simulink model "LQR"  (R2024b)
settings: Solver=ode45  StartTime=0.0  StopTime=10  RelTol=1e-3
values from neighbouring files (symbols this model uses):
  Beq = mot.B+(mld.Bh)/((gbox.N)^2)    [LQR_code.m]
  deltafil = 2^(-0.5)    (= 0.707106781187)    [LQR_code.m]    (also in PID_Luca.m)
  Jb = 1.4e-3    (= 0.0014)    [Elastic_parameters_estimation.m]
  K = acker(Aprime,Bprime,poles)    [LQR_code.m]
  Klqr1 = lqry(sysG,1,r2)    [LQR_code.m]
  Nu = N(5)    [LQR_code.m]
  Nx = [N(1);N(2);N(3);N(4)]    [LQR_code.m]
  omegac = 2*pi*50    (= 314.159265359)    [LQR_code.m]    (also in PID_Luca.m)
  Req = sens.curr.Rs+mot.R    [LQR_code.m]
undefined symbols (not defined in the file or in its folder): Bb, daq, degs2rpm, drv, gbox, Jeq_hat, k_drv, Ke, Kt, mot, pulse2deg, rads2rpm, rpm2rads, sens, T_drv, tau_sf
settings Model: Creator=lucag  LastModifiedBy=galeazzolu

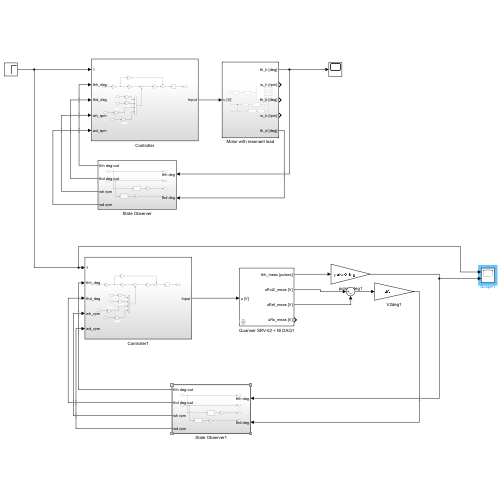
[thumbnail: Simulink's stored preview of the top-level diagram]
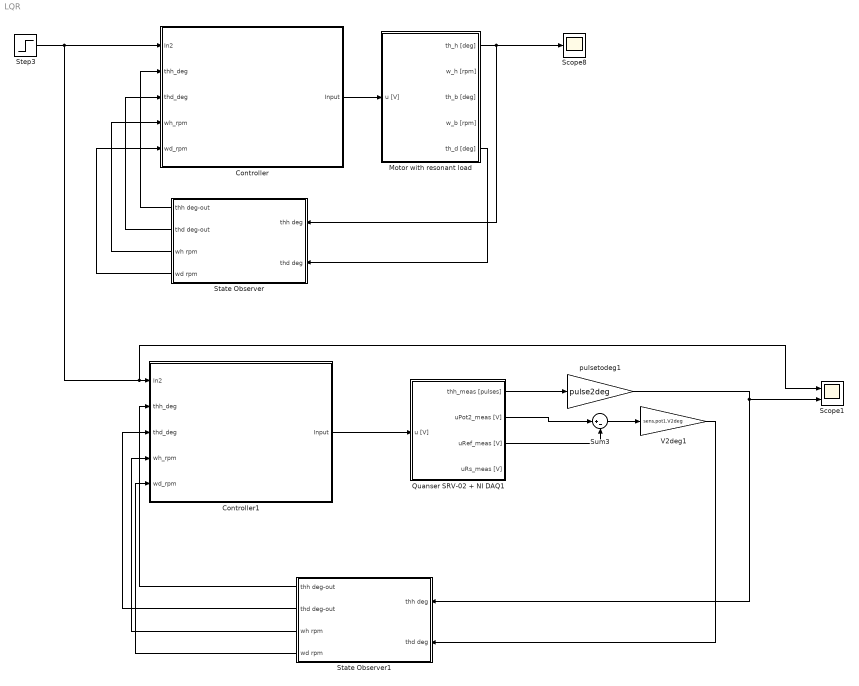
== system LQR ==
  Controller : Subsystem
  Controller1 : Subsystem
  Motor with resonant load : Subsystem
  Quanser SRV-02 + NI DAQ1 : Subsystem  mask(Quanser SRV-02 (with resonant load) + NI DAQ){Ts=0.001, fricType=Coulomb + viscous, lockShaft=off, beamInitPos=10}
      mask prompts: Ts "NI DAQ Sample Time:"; fricType "Friction model"; lockShaft "Lock motor shaft"; beamInitPos "Beam initial position [deg]:"
      mask help: Quanser SRV-02 (with resonant load) + NI DAQ model.
      mask init:
      | %%
      | % Riccardo Antonello (riccardo.antonello@unipd.it)
      | %
      | % April 28, 2020
      | %
      | % Dept. of Information Engineering, University of Padova
      | %
      | 
      | %%  Conversion gains
      | deg2rad = pi/180;                   %   [deg]   -> [rad]
      | rad2deg = 180/pi;                   %   [rad]   -> [deg]
      | 
      | 
      | %%  Sensors data
      | 
      | %   shunt resistor
      | sens.curr.Rs = 0.5;   
      | 
      | %   Hewlett-Packard HEDS-5540#A06 optical encoder
      | sens.enc.ppr = 500*4;                                                   %   pulses per rotation
      | sens.enc.pulse2deg = 360/sens.enc.ppr;                                  %   [pulses] -> [deg]
      | sens.enc.pulse2rad = 2*pi/sens.enc.ppr;                                 %   [pulses] -> [rad]
      | sens.enc.deg2pulse = sens.enc.ppr/360;                                  %   [deg] -> [pulses]
      | sens.enc.rad2pulse = sens.enc.ppr/2/pi;                                 %   [rad] -> [pulses]
      | 
      | %   potentiometer 2 (Spectrol 357-0-0-103) - installed on hub
      | sens.pot2.range.R      = 10e3;                                          %   ohmic value range 
      | sens.pot2.range.V      = 5;                                             %   voltage range
      | sens.pot2.range.th_deg = 340;                                           %   angle range [deg]
      | sens.pot2.range.th     = sens.pot2.range.th_deg * deg2rad;              %   angle range [rad]                           
      | sens.pot2.deg2V        = sens.pot2.range.V / sens.pot2.range.th_deg;    %   sensitivity [V/deg]
      | sens.pot2.rad2V        = sens.pot2.range.V / sens.pot2.range.th;        %   sensitivity [V/rad]
      | sens.pot2.V2deg        = 1/sens.pot2.deg2V;                             %   conversion gain [V] -> [deg]
      | sens.pot2.V2rad        = 1/sens.pot2.rad2V;                             %   conversion gain [V] -> [rad]
      | sens.pot2.noise.var    = 3.5e-7;                                        %   out noise variance [V^2]
      | 
      | 
      | %%  Data acquisition board (daq) data
      | 
      | %   NI PCI-6221 DAC data
      | daq.dac.bits = 16;                                  %   resolution (bits)
      | daq.dac.fs   = 10;                                  %   full scale 
      | daq.dac.q    = 2*daq.dac.fs/(2^daq.dac.bits-1);     %	quantization
      | 
      | %   NI PCI-6221 ADC data
      | daq.adc.bits = 16;                                  %   resolution (bits)
      | daq.adc.fs   = 10;                                  %   full scale (as set in SLDRT Analog Input block)
      | daq.adc.q    = 2*daq.adc.fs/(2^daq.adc.bits-1);     %   quantization   
      | 
      | 
      | %%  Set beam initial position
      | % SRV02Handle = find_system(gcb, ...
      | %     'LookUnderMasks', 'on', ...
      | %     'FindAll', 'on', ...
      | %     'FollowLinks', 'on', ...
      | %     'SearchDepth', '1', ...
      | %     'BlockType', 'ModelReference', ...
      | %     'Name', 'Quanser SRV-02');
      | %
      | % %get_param(SRV02Handle, 'InstanceParameters')
      | % InstanceParams = get_param(SRV02Handle, 'InstanceParameters');
      | % for k = 1:length(InstanceParams)
      | %     if strcmp(InstanceParams(k).Name, 'thb0')
      | %         if lockShaft
      | %             InstanceParams(k).Value = sprintf('%f', beamInitPos);
      | %         else
      | %             InstanceParams(k).Value = sprintf('%f', 0);    
      | %         end
      | %         set_param(SRV02Handle, 'InstanceParameters', InstanceParams);
      | %         break;
      | %     end
      | % end
      | 
      | if lockShaft
      |     thb0 = beamInitPos;
      | else
      |     thb0 = 0;    
      | end
      | 
      | 
      | %%  Mask initialization
      | if lockShaft
      |     
      |     %   find Inport handle
      |     InPortHandle = find_system(gcb, ...
      |         'LookUnderMasks', 'on', ...
      |         'FindAll', 'on', ...
      |         'FollowLinks', 'on', ...
      |         'SearchDepth', '1', ...
      |         'BlockType', 'Inport', ...
      |         'Name', 'u [V]');
      |     
      |     if ~isempty(InPortHandle)
      |     
      |         %   find DAC handle
      |         DACHandle = find_system(gcb, ...
      |             'LookUnderMasks', 'on', ...
      |             'FindAll', 'on', ...
      |             'FollowLinks', 'on', ...
      |             'SearchDepth', '1', ...
      |             'BlockType', 'SubSystem', ...
      |             'Name', 'DAC');  
      | 
      |         %   remove Inport output connection   
      |         InportConn = get_param(InPortHandle, 'PortConnectivity');
      |         delete_line(gcb, InportConn.Position);
      | 
      |         %   remove Inport block
      |         delete_block(InPortHandle);
      | 
      |         %   add Constant block
      |         ConstantHandle = add_block( ...
      |             'simulink/Sources/Constant', [gcb, '/u [V]'], ...
      |             'Position', [20   -37    50   -23], ...
      |             'Value', '0');
      | 
      |         %   connect Constant to DAC block
      |         DACPortHandles = get_param(DACHandle, 'PortHandles');
      |         ConstantPortHandles = get_param(ConstantHandle, 'PortHandles');
      |         add_line(gcb, ConstantPortHandles.Outport(1), DACPortHandles.Inport(1));
      |     
      |     end
      |     
      | else
      |     
      |     %   find Constant handle
      |     ConstantHandle = find_system(gcb, ...
      |         'LookUnderMasks', 'on', ...
      |         'FindAll', 'on', ...
      |         'FollowLinks', 'on', ...
      |         'SearchDepth', '1', ...
      |         'BlockType', 'Constant', ...
      |         'Name', 'u [V]');
      |     
      |     if ~isempty(ConstantHandle)
      |     
      |         %   find DAC handle
      |         DACHandle = find_system(gcb, ...
      |             'LookUnderMasks', 'on', ...
      |             'FindAll', 'on', ...
      |             'FollowLinks', 'on', ...
      |             'SearchDepth', '1', ...
      |             'BlockType', 'SubSystem', ...
      |             'Name', 'DAC');  
      |  
      |         %   remove Constant output connection   
      |         ConstantConn = get_param(ConstantHandle, 'PortConnectivity');
      |         delete_line(gcb, ConstantConn.Position);
      | 
      |         %   remove Inport block
      |         delete_block(ConstantHandle);   
      | 
      |         %   add Inport block
      |         InportHandle = add_block( ...
      |             'simulink/Sources/In1', [gcb, '/u [V]'], ...
      |             'Position', [20   -37    50   -23], ...
      |             'Port', '1');
      | 
      |         %   connect Constant to DAC block
      |         DACPortHandles = get_param(DACHandle, 'PortHandles');
      |         InportPortHandles = get_param(InportHandle, 'PortHandles');
      |         add_line(gcb, InportPortHandles.Outport(1), DACPortHandles.Inport(1));
      |     
      |      end
      |     
      | end
      mask Help:
      | Riccardo Antonello (antonello@dei.unipd.it)
      | 
      | April 28, 2020
      | 
      | Dept. of Information Engineering, University of Padova
      mask TypeOptions fricType: Coulomb + viscous | Karnopp
      mask Callback lockShaft:
      | %   get status of check box
      | lockShaft = get_param(gcb, 'lockShaft');
      | 
      | %   get current value of MaskVisibilities property
      | maskVisibilities = get_param(gcb, 'MaskVisibilities');
      | 
      | %   set visibility of the dialog box element
      | if strcmp(lockShaft, 'on')
      |     maskVisibilities{4} = 'on';
      | else
      |     maskVisibilities{4} = 'off';
      | end
      | 
      | % Set the 'MaskVisibilities' property for each parameter in mask
      | set_param( gcb, 'MaskVisibilities', maskVisibilities);
  Scope1 : Scope  NumInputPorts=2
  Scope8 : Scope
  State Observer : Subsystem
  State Observer1 : Subsystem
  Step3 : Step  Time=0  After=50  SampleTime=0.001  ZeroCross=off
  Sum3 : Sum  Inputs=|+-
  V2deg1 : Gain  Gain=sens.pot1.V2deg
  pulsetodeg1 : Gain  Gain=pulse2deg
  wires:
  Controller/1(Input) -> Motor with resonant load/1(u [V])
  Motor with resonant load/1(th_h [deg]) -> Scope8/1, State Observer/1(thh deg)
  Motor with resonant load/5(th_d [deg]) -> State Observer/2(thd deg)
  State Observer/1(thh deg-out) -> Controller/2(thh_deg)
  State Observer/2(thd deg-out) -> Controller/3(thd_deg)
  State Observer/3(wh rpm) -> Controller/4(wh_rpm)
  State Observer/4(wd rpm) -> Controller/5(wd_rpm)
  Step3/1 -> Scope1/1, Controller1/1(In2), Controller/1(In2)
  Quanser SRV-02 + NI DAQ1/3(uRef_meas [V]) -> Sum3/2
  Quanser SRV-02 + NI DAQ1/1(thh_meas [pulses]) -> pulsetodeg1/1
  Sum3/1 -> V2deg1/1
  Quanser SRV-02 + NI DAQ1/2(uPot2_meas [V]) -> Sum3/1
  pulsetodeg1/1 -> Scope1/2, State Observer1/1(thh deg)
  V2deg1/1 -> State Observer1/2(thd deg)
  State Observer1/1(thh deg-out) -> Controller1/2(thh_deg)
  State Observer1/2(thd deg-out) -> Controller1/3(thd_deg)
  State Observer1/3(wh rpm) -> Controller1/4(wh_rpm)
  State Observer1/4(wd rpm) -> Controller1/5(wd_rpm)
  Controller1/1(Input) -> Quanser SRV-02 + NI DAQ1/1(u [V])

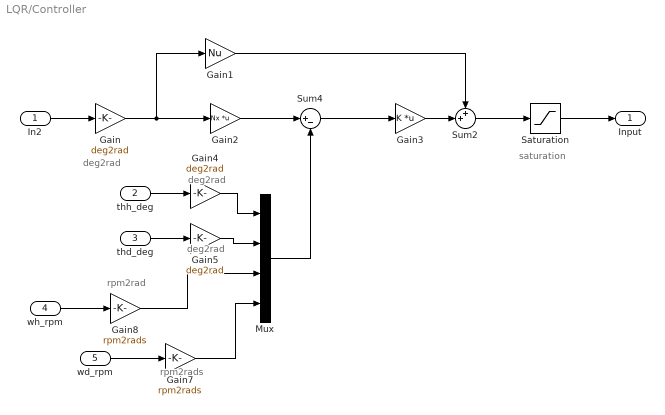
== system LQR/Controller ==
  note: rpm2rad
  note: deg2rad
  note: deg2rad
  note: deg2rad
  note: saturation
  note: rpm2rads
  In2 : Inport  PortDimensions=1
  thh_deg : Inport  Port=2
  thd_deg : Inport  Port=3
  wh_rpm : Inport  Port=4
  wd_rpm : Inport  Port=5
  Gain : Gain  Gain=deg2rad
  Gain1 : Gain  Gain=Nu
  Gain2 : Gain  Gain=Nx  Multiplication=Matrix(K*u)
  Gain3 : Gain  Gain=K  Multiplication=Matrix(K*u)
  Gain4 : Gain  Gain=deg2rad
  Gain5 : Gain  Gain=deg2rad
  Gain7 : Gain  Gain=rpm2rads
  Gain8 : Gain  Gain=rpm2rads
  Mux : Mux
  Saturation : Saturate  UpperLimit=12  LowerLimit=-12  ZeroCross=off
  Sum2 : Sum  Inputs=++|
  Sum4 : Sum  Inputs=|+-
  Input : Outport  PortDimensions=1
  wires:
  thd_deg/1 -> Gain5/1
  Gain4/1 -> Mux/1
  thh_deg/1 -> Gain4/1
  Gain5/1 -> Mux/2
  Gain/1 -> Gain1/1, Gain2/1
  Saturation/1 -> Input/1
  Sum2/1 -> Saturation/1
  Gain1/1 -> Sum2/1
  Gain3/1 -> Sum2/2
  Gain2/1 -> Sum4/1
  Mux/1 -> Sum4/2
  In2/1 -> Gain/1
  Sum4/1 -> Gain3/1
  Gain7/1 -> Mux/4
  wh_rpm/1 -> Gain8/1
  Gain8/1 -> Mux/3
  wd_rpm/1 -> Gain7/1

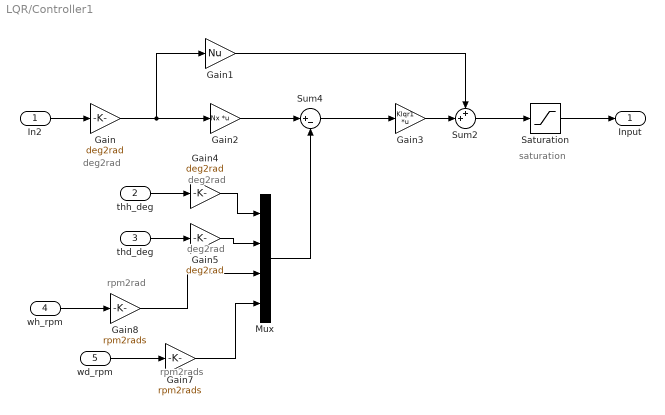
== system LQR/Controller1 ==
  note: rpm2rad
  note: deg2rad
  note: deg2rad
  note: deg2rad
  note: saturation
  note: rpm2rads
  In2 : Inport  PortDimensions=1
  thh_deg : Inport  Port=2
  thd_deg : Inport  Port=3
  wh_rpm : Inport  Port=4
  wd_rpm : Inport  Port=5
  Gain : Gain  Gain=deg2rad
  Gain1 : Gain  Gain=Nu
  Gain2 : Gain  Gain=Nx  Multiplication=Matrix(K*u)
  Gain3 : Gain  Gain=Klqr1  Multiplication=Matrix(K*u)
  Gain4 : Gain  Gain=deg2rad
  Gain5 : Gain  Gain=deg2rad
  Gain7 : Gain  Gain=rpm2rads
  Gain8 : Gain  Gain=rpm2rads
  Mux : Mux
  Saturation : Saturate  UpperLimit=12  LowerLimit=-12  ZeroCross=off
  Sum2 : Sum  Inputs=++|
  Sum4 : Sum  Inputs=|+-
  Input : Outport  PortDimensions=1
  wires:
  thd_deg/1 -> Gain5/1
  Gain4/1 -> Mux/1
  thh_deg/1 -> Gain4/1
  Gain5/1 -> Mux/2
  Gain/1 -> Gain1/1, Gain2/1
  Saturation/1 -> Input/1
  Sum2/1 -> Saturation/1
  Gain1/1 -> Sum2/1
  Gain3/1 -> Sum2/2
  Gain2/1 -> Sum4/1
  Mux/1 -> Sum4/2
  In2/1 -> Gain/1
  Sum4/1 -> Gain3/1
  Gain7/1 -> Mux/4
  wh_rpm/1 -> Gain8/1
  Gain8/1 -> Mux/3
  wd_rpm/1 -> Gain7/1

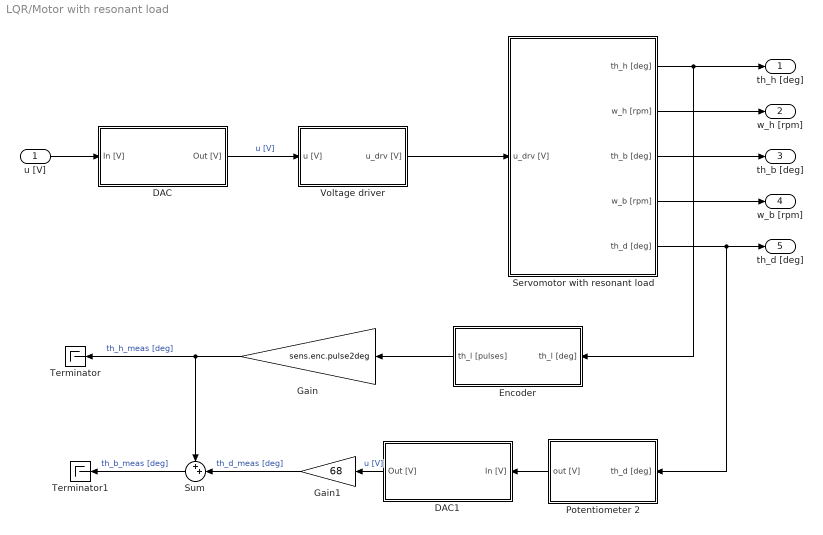
== system LQR/Motor with resonant load ==
  u [V] : Inport
  DAC : Subsystem
  DAC1 : Subsystem
  Encoder : Subsystem
  Gain : Gain  Gain=sens.enc.pulse2deg
  Gain1 : Gain  Gain=68
  Potentiometer 2 : Subsystem
  Servomotor with resonant load : Subsystem
  Sum : Sum  Inputs=++|
  Terminator : Terminator
  Terminator1 : Terminator
  Voltage driver : Subsystem
  th_h [deg] : Outport
  w_h [rpm] : Outport  Port=2
  th_b [deg] : Outport  Port=3
  w_b [rpm] : Outport  Port=4
  th_d [deg] : Outport  Port=5
  wires:
  Encoder/1(th_l [pulses]) -> Gain/1
  u [V]/1 -> DAC/1(In [V])
  DAC/1(Out [V]) -> Voltage driver/1(u [V])  "u [V]"
  Voltage driver/1(u_drv [V]) -> Servomotor with resonant load/1(u_drv [V])
  Servomotor with resonant load/1(th_h [deg]) -> Encoder/1(th_l [deg]), th_h [deg]/1
  Servomotor with resonant load/2(w_h [rpm]) -> w_h [rpm]/1
  Servomotor with resonant load/3(th_b [deg]) -> th_b [deg]/1
  Servomotor with resonant load/4(w_b [rpm]) -> w_b [rpm]/1
  Servomotor with resonant load/5(th_d [deg]) -> Potentiometer 2/1(th_d [deg]), th_d [deg]/1
  Gain/1 -> Terminator/1, Sum/1  "th_h_meas [deg]"
  Potentiometer 2/1(out [V]) -> DAC1/1(In [V])
  DAC1/1(Out [V]) -> Gain1/1  "u [V]"
  Gain1/1 -> Sum/2  "th_d_meas [deg]"
  Sum/1 -> Terminator1/1  "th_b_meas [deg]"

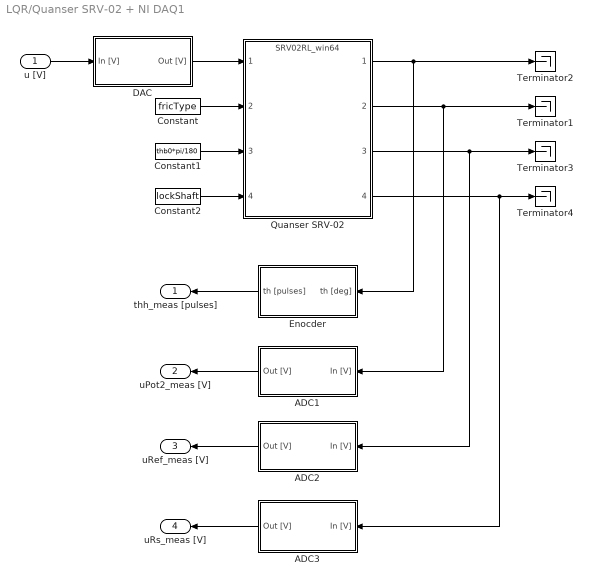
== system LQR/Quanser SRV-02 + NI DAQ1 ==
  u [V] : Inport
  ADC1 : Subsystem
  ADC2 : Subsystem
  ADC3 : Subsystem
  Constant : Constant  Value=fricType
  Constant1 : Constant  Value=thb0*pi/180  SampleTime=Inf
  Constant2 : Constant  Value=lockShaft  SampleTime=Inf
  DAC : Subsystem
  Enocder : Subsystem
  Quanser SRV-02 : ModelReference  ModelNameDialog=SRV02RL_win64.slxp  ModelReferenceVersion=1.76  CopyOfModelProtected=on
  Terminator{1..4} (4 alike) : Terminator
  thh_meas [pulses] : Outport
  uPot2_meas [V] : Outport  Port=2
  uRef_meas [V] : Outport  Port=3
  uRs_meas [V] : Outport  Port=4
  wires:
  Enocder/1(th [pulses]) -> thh_meas [pulses]/1
  ADC3/1(Out [V]) -> uRs_meas [V]/1
  DAC/1(Out [V]) -> Quanser SRV-02/1
  Quanser SRV-02/2 -> ADC1/1(In [V]), Terminator1/1
  Quanser SRV-02/1 -> Terminator2/1, Enocder/1(th [deg])
  Constant/1 -> Quanser SRV-02/2
  Quanser SRV-02/3 -> ADC2/1(In [V]), Terminator3/1
  ADC1/1(Out [V]) -> uPot2_meas [V]/1
  Constant1/1 -> Quanser SRV-02/3
  Constant2/1 -> Quanser SRV-02/4
  Quanser SRV-02/4 -> ADC3/1(In [V]), Terminator4/1
  ADC2/1(Out [V]) -> uRef_meas [V]/1
  u [V]/1 -> DAC/1(In [V])

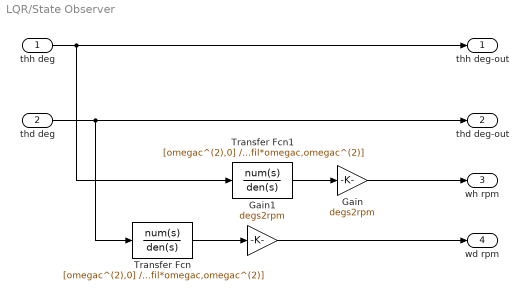
== system LQR/State Observer ==
  thh deg : Inport
  thd deg : Inport  Port=2
  Gain : Gain  Gain=degs2rpm
  Gain1 : Gain  Gain=degs2rpm
  Transfer Fcn : TransferFcn  Numerator=[omegac^(2),0]  Denominator=[1,2*deltafil*omegac,omegac^(2)]
  Transfer Fcn1 : TransferFcn  Numerator=[omegac^(2),0]  Denominator=[1,2*deltafil*omegac,omegac^(2)]
  thh deg-out : Outport
  thd deg-out : Outport  Port=2
  wh rpm : Outport  Port=3
  wd rpm : Outport  Port=4
  wires:
  thh deg/1 -> Transfer Fcn1/1, thh deg-out/1
  thd deg/1 -> Transfer Fcn/1, thd deg-out/1
  Transfer Fcn1/1 -> Gain/1
  Gain/1 -> wh rpm/1
  Gain1/1 -> wd rpm/1
  Transfer Fcn/1 -> Gain1/1

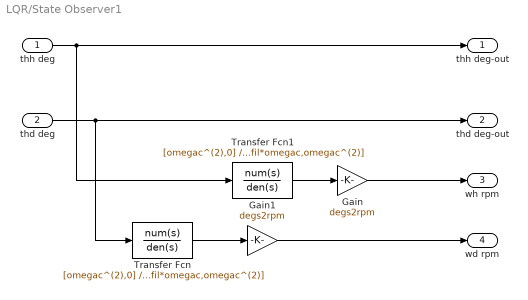
== system LQR/State Observer1 ==
  thh deg : Inport
  thd deg : Inport  Port=2
  Gain : Gain  Gain=degs2rpm
  Gain1 : Gain  Gain=degs2rpm
  Transfer Fcn : TransferFcn  Numerator=[omegac^(2),0]  Denominator=[1,2*deltafil*omegac,omegac^(2)]
  Transfer Fcn1 : TransferFcn  Numerator=[omegac^(2),0]  Denominator=[1,2*deltafil*omegac,omegac^(2)]
  thh deg-out : Outport
  thd deg-out : Outport  Port=2
  wh rpm : Outport  Port=3
  wd rpm : Outport  Port=4
  wires:
  thh deg/1 -> Transfer Fcn1/1, thh deg-out/1
  thd deg/1 -> Transfer Fcn/1, thd deg-out/1
  Transfer Fcn1/1 -> Gain/1
  Gain/1 -> wh rpm/1
  Gain1/1 -> wd rpm/1
  Transfer Fcn/1 -> Gain1/1

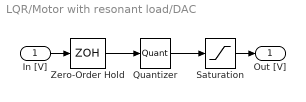
== system LQR/Motor with resonant load/DAC ==
  In [V] : Inport
  Quantizer : Quantizer  QuantizationInterval=daq.dac.q
  Saturation : Saturate  UpperLimit=daq.dac.fs  LowerLimit=-daq.dac.fs
  Zero-Order Hold : ZeroOrderHold  SampleTime=0.001
  Out [V] : Outport
  wires:
  Saturation/1 -> Out [V]/1
  Zero-Order Hold/1 -> Quantizer/1
  Quantizer/1 -> Saturation/1
  In [V]/1 -> Zero-Order Hold/1

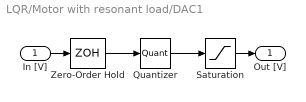
== system LQR/Motor with resonant load/DAC1 ==
  In [V] : Inport
  Quantizer : Quantizer  QuantizationInterval=daq.dac.q
  Saturation : Saturate  UpperLimit=daq.dac.fs  LowerLimit=-daq.dac.fs
  Zero-Order Hold : ZeroOrderHold  SampleTime=1e-3
  Out [V] : Outport
  wires:
  In [V]/1 -> Zero-Order Hold/1
  Quantizer/1 -> Saturation/1
  Zero-Order Hold/1 -> Quantizer/1
  Saturation/1 -> Out [V]/1

== system LQR/Motor with resonant load/Encoder ==
  th_l [deg] : Inport
  Gain : Gain  Gain=1/sens.enc.pulse2deg
  Quantizer : Quantizer  QuantizationInterval=sens.enc.pulse2deg
  Zero-Order Hold : ZeroOrderHold  SampleTime=1e-3
  th_l [pulses] : Outport
  wires:
  th_l [deg]/1 -> Zero-Order Hold/1
  Quantizer/1 -> Gain/1
  Zero-Order Hold/1 -> Quantizer/1
  Gain/1 -> th_l [pulses]/1

== system LQR/Motor with resonant load/Potentiometer 2 ==
  th_d [deg] : Inport
  Gain1 : Gain  Gain=0.014706
  Random Number : RandomNumber  Variance=sens.pot2.noise.var  SampleTime=1e-3
  Sum : Sum  Inputs=++|
  out [V] : Outport
  wires:
  Gain1/1 -> Sum/2
  th_d [deg]/1 -> Gain1/1
  Random Number/1 -> Sum/1
  Sum/1 -> out [V]/1

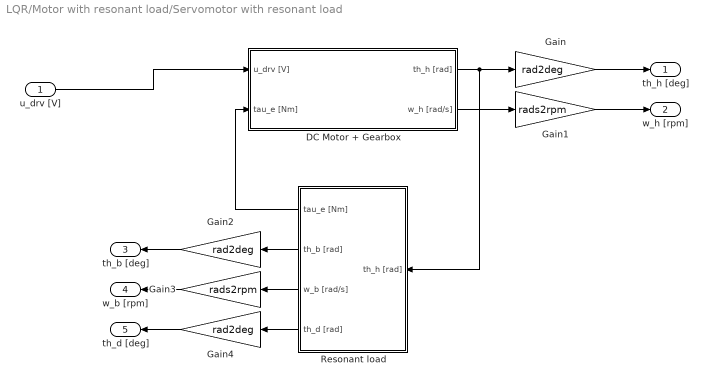
== system LQR/Motor with resonant load/Servomotor with resonant load ==
  u_drv [V] : Inport
  DC Motor + Gearbox : Subsystem
  Gain : Gain  Gain=rad2deg
  Gain1 : Gain  Gain=rads2rpm
  Gain2 : Gain  Gain=rad2deg
  Gain3 : Gain  Gain=rads2rpm
  Gain4 : Gain  Gain=rad2deg
  Resonant load : Subsystem
  th_h [deg] : Outport
  w_h [rpm] : Outport  Port=2
  th_b [deg] : Outport  Port=3
  w_b [rpm] : Outport  Port=4
  th_d [deg] : Outport  Port=5
  wires:
  Resonant load/1(tau_e [Nm]) -> DC Motor + Gearbox/2(tau_e [Nm])
  Gain4/1 -> th_d [deg]/1
  Gain2/1 -> th_b [deg]/1
  Resonant load/2(th_b [rad]) -> Gain2/1
  DC Motor + Gearbox/2(w_h [rad/s]) -> Gain1/1
  DC Motor + Gearbox/1(th_h [rad]) -> Gain/1, Resonant load/1(th_h [rad])
  Resonant load/3(w_b [rad/s]) -> Gain3/1
  Gain1/1 -> w_h [rpm]/1
  Resonant load/4(th_d [rad]) -> Gain4/1
  Gain/1 -> th_h [deg]/1
  Gain3/1 -> w_b [rpm]/1
  u_drv [V]/1 -> DC Motor + Gearbox/1(u_drv [V])

== system LQR/Motor with resonant load/Voltage driver ==
  u [V] : Inport
  Driver dynamics : TransferFcn  Numerator=[k_drv]  Denominator=[T_drv 1]
  Driver saturation : Saturate  UpperLimit=drv.outmax  LowerLimit=-drv.outmax
  u_drv [V] : Outport
  wires:
  Driver dynamics/1 -> Driver saturation/1
  Driver saturation/1 -> u_drv [V]/1
  u [V]/1 -> Driver dynamics/1

== system LQR/Quanser SRV-02 + NI DAQ1/ADC1 ==
  In [V] : Inport
  ADC quantization : Quantizer  QuantizationInterval=daq.adc.q
  ADC sampling : ZeroOrderHold  SampleTime=Ts
  ADC saturation : Saturate  UpperLimit=daq.adc.fs  LowerLimit=-daq.adc.fs
  Out [V] : Outport
  wires:
  ADC saturation/1 -> Out [V]/1
  ADC sampling/1 -> ADC quantization/1
  In [V]/1 -> ADC sampling/1
  ADC quantization/1 -> ADC saturation/1

== system LQR/Quanser SRV-02 + NI DAQ1/ADC2 ==
  In [V] : Inport
  ADC quantization : Quantizer  QuantizationInterval=daq.adc.q
  ADC sampling : ZeroOrderHold  SampleTime=Ts
  ADC saturation : Saturate  UpperLimit=daq.adc.fs  LowerLimit=-daq.adc.fs
  Out [V] : Outport
  wires:
  ADC quantization/1 -> ADC saturation/1
  In [V]/1 -> ADC sampling/1
  ADC sampling/1 -> ADC quantization/1
  ADC saturation/1 -> Out [V]/1

== system LQR/Quanser SRV-02 + NI DAQ1/ADC3 ==
  In [V] : Inport
  Quantizer : Quantizer  QuantizationInterval=daq.adc.q
  Saturation : Saturate  UpperLimit=daq.adc.fs  LowerLimit=-daq.adc.fs
  Zero-Order Hold : ZeroOrderHold  SampleTime=Ts
  Out [V] : Outport
  wires:
  Saturation/1 -> Out [V]/1
  In [V]/1 -> Zero-Order Hold/1
  Quantizer/1 -> Saturation/1
  Zero-Order Hold/1 -> Quantizer/1

== system LQR/Quanser SRV-02 + NI DAQ1/DAC ==
  In [V] : Inport
  Quantizer : Quantizer  QuantizationInterval=daq.dac.q
  Saturation : Saturate  UpperLimit=daq.dac.fs  LowerLimit=-daq.dac.fs
  Zero-Order Hold : ZeroOrderHold  SampleTime=Ts
  Out [V] : Outport
  wires:
  Quantizer/1 -> Saturation/1
  In [V]/1 -> Zero-Order Hold/1
  Zero-Order Hold/1 -> Quantizer/1
  Saturation/1 -> Out [V]/1

== system LQR/Quanser SRV-02 + NI DAQ1/Enocder ==
  th [deg] : Inport
  Quantizer : Quantizer  QuantizationInterval=sens.enc.pulse2deg
  Zero-Order Hold : ZeroOrderHold  SampleTime=Ts
  deg2pulse : Gain  Gain=sens.enc.deg2pulse
  th [pulses] : Outport
  wires:
  Quantizer/1 -> deg2pulse/1
  th [deg]/1 -> Zero-Order Hold/1
  Zero-Order Hold/1 -> Quantizer/1
  deg2pulse/1 -> th [pulses]/1

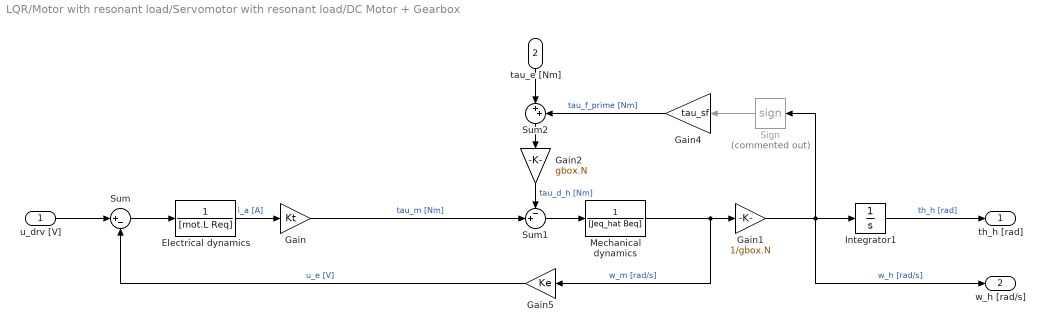
== system LQR/Motor with resonant load/Servomotor with resonant load/DC Motor + Gearbox ==
  u_drv [V] : Inport
  tau_e [Nm] : Inport  Port=2
  Electrical dynamics : TransferFcn  Denominator=[mot.L Req]
  Gain : Gain  Gain=Kt
  Gain1 : Gain  Gain=1/gbox.N
  Gain2 : Gain  Gain=gbox.N
  Gain4 : Gain  Gain=tau_sf
  Gain5 : Gain  Gain=Ke
  Integrator1 : Integrator
  Mechanical dynamics : TransferFcn  Denominator=[Jeq_hat Beq]
  Sign : Signum  Commented=on  ZeroCross=off
  Sum : Sum  Inputs=|+-
  Sum1 : Sum  Inputs=-+|
  Sum2 : Sum  Inputs=|++
  th_h [rad] : Outport
  w_h [rad/s] : Outport  Port=2
  wires:
  Integrator1/1 -> th_h [rad]/1  "th_h [rad]"
  Gain5/1 -> Sum/2  "u_e [V]"
  Gain1/1 -> Sign/1, w_h [rad/s]/1, Integrator1/1  "w_h [rad/s]"
  Electrical dynamics/1 -> Gain/1  "i_a [A]"
  Sign/1 -> Gain4/1
  Sum/1 -> Electrical dynamics/1
  Sum1/1 -> Mechanical dynamics/1
  Gain/1 -> Sum1/2  "tau_m [Nm]"
  Mechanical dynamics/1 -> Gain5/1, Gain1/1  "w_m [rad/s]"
  u_drv [V]/1 -> Sum/1
  Gain4/1 -> Sum2/2  "tau_f_prime [Nm]"
  Sum2/1 -> Gain2/1
  tau_e [Nm]/1 -> Sum2/1
  Gain2/1 -> Sum1/1  "tau_d_h [Nm]"

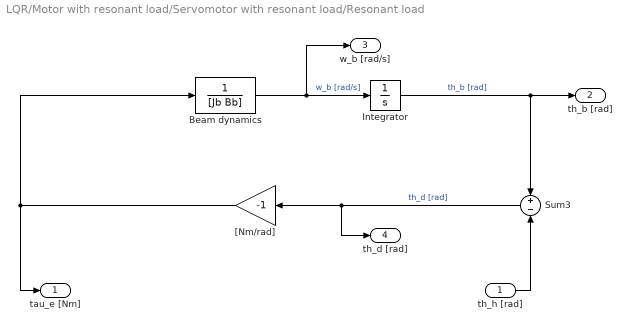
== system LQR/Motor with resonant load/Servomotor with resonant load/Resonant load ==
  th_h [rad] : Inport
  Beam dynamics : TransferFcn  Denominator=[Jb Bb]
  Integrator : Integrator
  Sum3 : Sum  Inputs=+|-
  "[Nm/rad]" : Gain  Gain=-1
  tau_e [Nm] : Outport
  th_b [rad] : Outport  Port=2
  w_b [rad/s] : Outport  Port=3
  th_d [rad] : Outport  Port=4
  wires:
  Integrator/1 -> th_b [rad]/1, Sum3/1  "th_b [rad]"
  "[Nm/rad]"/1 -> tau_e [Nm]/1, Beam dynamics/1
  Sum3/1 -> th_d [rad]/1, "[Nm/rad]"/1  "th_d [rad]"
  Beam dynamics/1 -> w_b [rad/s]/1, Integrator/1  "w_b [rad/s]"
  th_h [rad]/1 -> Sum3/2
